simulink model "messy_single_sensor"  (R2024b)
settings: Solver=VariableStepAuto  StartTime=0.0  StopTime=10.0  RelTol=1e-3
settings Model: Creator=giovanni  LastModifiedBy=giovanni
settings RTWCC: GPUComputeCapability=3.5

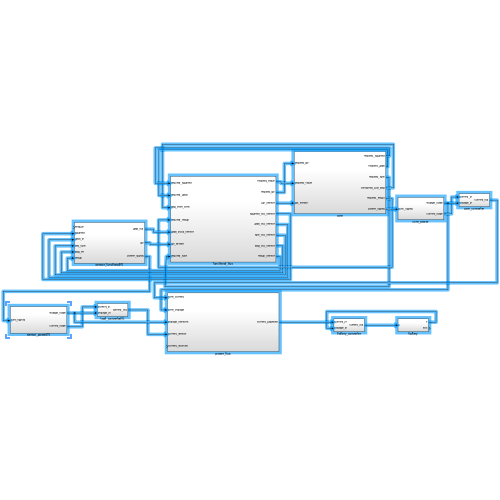
[thumbnail: Simulink's stored preview of the top-level diagram]
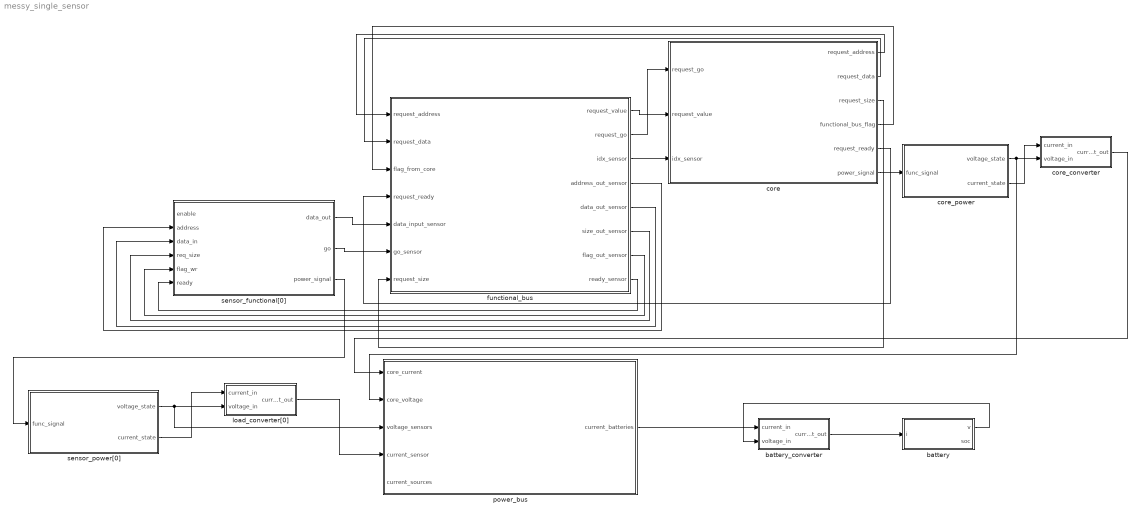
== system messy_single_sensor ==
  battery : Subsystem
  battery_converter : Subsystem
  core : Subsystem
  core_converter : Subsystem
  core_power : Subsystem
  functional_bus : Subsystem
  load_converter[0] : Subsystem
  power_bus : Subsystem
  sensor_functional[0] : Subsystem
  sensor_power[0] : Subsystem
  wires:
  core/4(functional_bus_flag) -> functional_bus/3(flag_from_core)
  functional_bus/6(size_out_sensor) -> sensor_functional[0]/4(req_size)
  sensor_power[0]/2(current_state) -> load_converter[0]/1(current_in)
  core/5(request_ready) -> functional_bus/4(request_ready)
  functional_bus/8(ready_sensor) -> sensor_functional[0]/6(ready)
  core_power/2(current_state) -> core_converter/1(current_in)
  sensor_functional[0]/2(go) -> functional_bus/6(go_sensor)
  sensor_functional[0]/3(power_signal) -> sensor_power[0]/1(func_signal)
  battery/1(v) -> battery_converter/2(voltage_in)
  sensor_functional[0]/1(data_out) -> functional_bus/5(data_input_sensor)
  core_power/1(voltage_state) -> core_converter/2(voltage_in), power_bus/2(core_voltage)
  core/2(request_data) -> functional_bus/2(request_data)
  sensor_power[0]/1(voltage_state) -> load_converter[0]/2(voltage_in), power_bus/3(voltage_sensors)
  power_bus/1(current_batteries) -> battery_converter/1(current_in)
  functional_bus/5(data_out_sensor) -> sensor_functional[0]/3(data_in)
  functional_bus/1(request_value) -> core/2(request_value)
  core/6(power_signal) -> core_power/1(func_signal)
  functional_bus/7(flag_out_sensor) -> sensor_functional[0]/5(flag_wr)
  core_converter/1(current_out) -> power_bus/1(core_current)
  functional_bus/2(request_go) -> core/1(request_go)
  functional_bus/3(idx_sensor) -> core/3(idx_sensor)
  battery_converter/1(current_out) -> battery/1(i)
  core/3(request_size) -> functional_bus/7(request_size)
  load_converter[0]/1(current_out) -> power_bus/4(current_sensor)
  core/1(request_address) -> functional_bus/1(request_address)
  functional_bus/4(address_out_sensor) -> sensor_functional[0]/2(address)

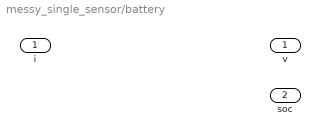
== system messy_single_sensor/battery ==
  i : Inport
  v : Outport
  soc : Outport  Port=2

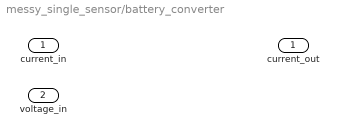
== system messy_single_sensor/battery_converter ==
  current_in : Inport
  voltage_in : Inport  Port=2
  current_out : Outport

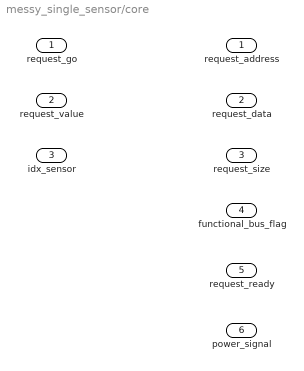
== system messy_single_sensor/core ==
  request_go : Inport
  request_value : Inport  Port=2
  idx_sensor : Inport  Port=3
  request_address : Outport
  request_data : Outport  Port=2
  request_size : Outport  Port=3
  functional_bus_flag : Outport  Port=4
  request_ready : Outport  Port=5
  power_signal : Outport  Port=6

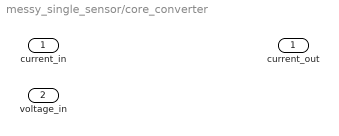
== system messy_single_sensor/core_converter ==
  current_in : Inport
  voltage_in : Inport  Port=2
  current_out : Outport

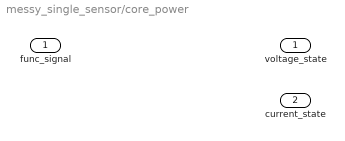
== system messy_single_sensor/core_power ==
  func_signal : Inport
  voltage_state : Outport
  current_state : Outport  Port=2

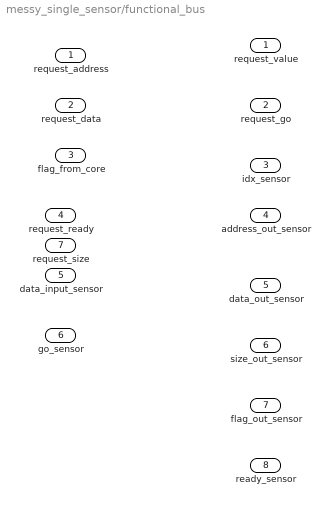
== system messy_single_sensor/functional_bus ==
  request_address : Inport
  request_data : Inport  Port=2
  flag_from_core : Inport  Port=3
  request_ready : Inport  Port=4
  data_input_sensor : Inport  Port=5
  go_sensor : Inport  Port=6
  request_size : Inport  Port=7
  request_value : Outport
  request_go : Outport  Port=2
  idx_sensor : Outport  Port=3
  address_out_sensor : Outport  Port=4
  data_out_sensor : Outport  Port=5
  size_out_sensor : Outport  Port=6
  flag_out_sensor : Outport  Port=7
  ready_sensor : Outport  Port=8

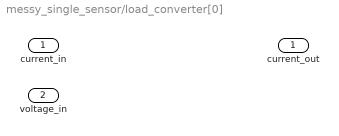
== system messy_single_sensor/load_converter[0] ==
  current_in : Inport
  voltage_in : Inport  Port=2
  current_out : Outport

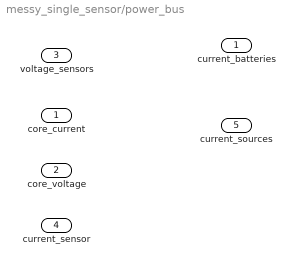
== system messy_single_sensor/power_bus ==
  core_current : Inport
  core_voltage : Inport  Port=2
  voltage_sensors : Inport  Port=3
  current_sensor : Inport  Port=4
  current_sources : Inport  Port=5
  current_batteries : Outport

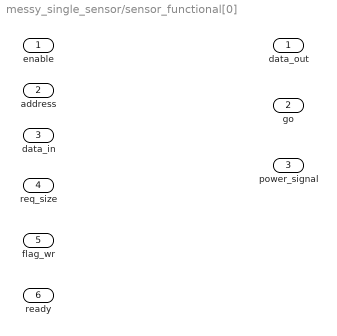
== system messy_single_sensor/sensor_functional[0] ==
  enable : Inport
  address : Inport  Port=2
  data_in : Inport  Port=3
  req_size : Inport  Port=4
  flag_wr : Inport  Port=5
  ready : Inport  Port=6
  data_out : Outport
  go : Outport  Port=2
  power_signal : Outport  Port=3

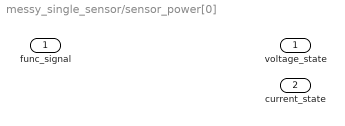
== system messy_single_sensor/sensor_power[0] ==
  func_signal : Inport
  voltage_state : Outport
  current_state : Outport  Port=2
